simulink model "dsm_l1_sim"  (Simulink 10.0)
settings: Solver=FixedStepDiscrete  StartTime=0.0  StopTime=1024  RelTol=1e-3  AbsTol=1e-6
undefined symbols (not defined in the file): a, b, c, g, Ts
settings Model: Creator=mimeiners  LastModifiedBy=ADMIN
settings SolverCC: AutoScaleAbsTol=off
settings DataIOCC: SignalLoggingSaveFormat=ModelDataLogs  SignalLoggingName=sigsOut
settings OptimizationCC: BooleanDataType=off  LifeSpan=auto
settings DebuggingCC: SaveWithParameterizedLinksMsg=none  SignalResolutionControl=TryResolveAllWithWarning  MultiTaskDSMMsg=warning  MultiTaskCondExecSysMsg=none  SFUnexpectedBacktrackingDiag=error  SFNoUnconditionalDefaultTransitionDiag=error  SFExecutionAtInitializationDiag=warning
settings HardwareCC: TargetUnknown=on
settings RTWCC: TemplateMakefile=grt_vc.tmf
settings CodeAppCC: StateflowObjectComments=off
settings ConfigComp: CovExternalEMLEnable=off

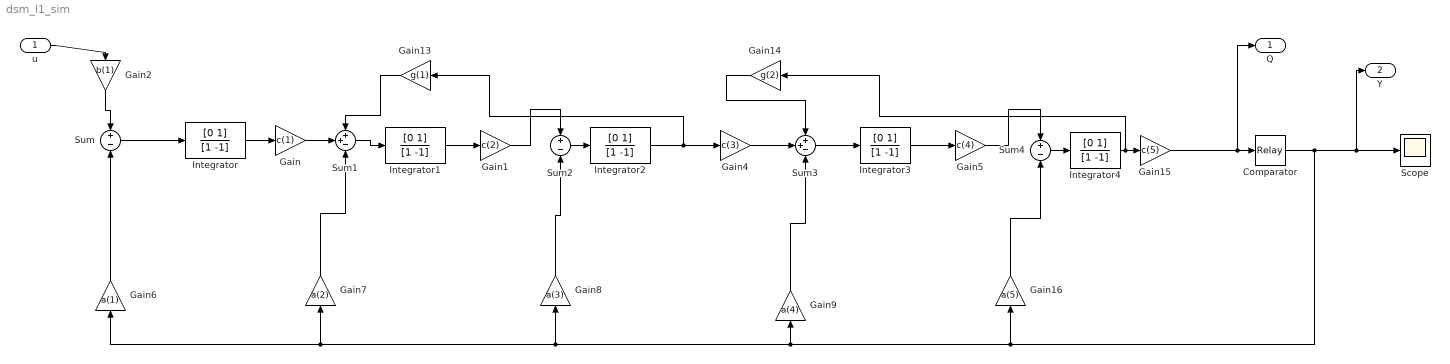
== system dsm_l1_sim ==
  "u " : Inport
  Comparator : Relay  OffOutputValue=-1
  Gain : Gain  Gain=c(1)
  Gain1 : Gain  Gain=c(2)
  Gain13 : Gain  Gain=g(1)
  Gain14 : Gain  Gain=g(2)
  Gain15 : Gain  Gain=c(5)
  Gain16 : Gain  Gain=a(5)
  Gain2 : Gain  Gain=b(1)
  Gain4 : Gain  Gain=c(3)
  Gain5 : Gain  Gain=c(4)
  Gain6 : Gain  Gain=a(1)
  Gain7 : Gain  Gain=a(2)
  Gain8 : Gain  Gain=a(3)
  Gain9 : Gain  Gain=a(4)
  Integrator{,1..4} (5 alike) : DiscreteFilter  Numerator=[0 1]  Denominator=[1 -1]  SampleTime=Ts
  Scope : Scope
  Sum : Sum  Inputs=+-  SaturateOnIntegerOverflow=on  InputSameDT=on  OutDataTypeStr=Inherit: Same as first input
  Sum1 : Sum  Inputs=++-  SaturateOnIntegerOverflow=on  InputSameDT=on  OutDataTypeStr=Inherit: Same as first input
  Sum2 : Sum  Inputs=+-  SaturateOnIntegerOverflow=on  InputSameDT=on  OutDataTypeStr=Inherit: Same as first input
  Sum3 : Sum  Inputs=++-  SaturateOnIntegerOverflow=on  InputSameDT=on  OutDataTypeStr=Inherit: Same as first input
  Sum4 : Sum  Inputs=+-  SaturateOnIntegerOverflow=on  InputSameDT=on  OutDataTypeStr=Inherit: Same as first input
  Q : Outport  VectorParamsAs1DForOutWhenUnconnected=off
  Y : Outport  Port=2  VectorParamsAs1DForOutWhenUnconnected=off
  wires:
  Sum/1 -> Integrator/1
  Integrator1/1 -> Gain1/1
  Sum2/1 -> Integrator2/1
  Integrator/1 -> Gain/1
  Sum1/1 -> Integrator1/1
  Sum3/1 -> Integrator3/1
  Integrator3/1 -> Gain5/1
  "u "/1 -> Gain2/1
  Comparator/1 -> Y/1, Scope/1, Gain16/1, Gain6/1, Gain7/1, Gain8/1, Gain9/1
  Sum4/1 -> Integrator4/1
  Gain2/1 -> Sum/1
  Gain6/1 -> Sum/2
  Gain13/1 -> Sum1/1
  Integrator2/1 -> Gain13/1, Gain4/1
  Integrator4/1 -> Gain14/1, Gain15/1
  Gain15/1 -> Q/1, Comparator/1
  Gain/1 -> Sum1/2
  Gain7/1 -> Sum1/3
  Gain1/1 -> Sum2/1
  Gain14/1 -> Sum3/1
  Gain4/1 -> Sum3/2
  Gain9/1 -> Sum3/3
  Gain5/1 -> Sum4/1
  Gain16/1 -> Sum4/2
  Gain8/1 -> Sum2/2
